simulink model "Lateral"  (R2020a)
settings: Solver=VariableStepAuto  StartTime=0.0  StopTime=5  RelTol=1e-3
settings Model: Creator=hp  LastModifiedBy=hp

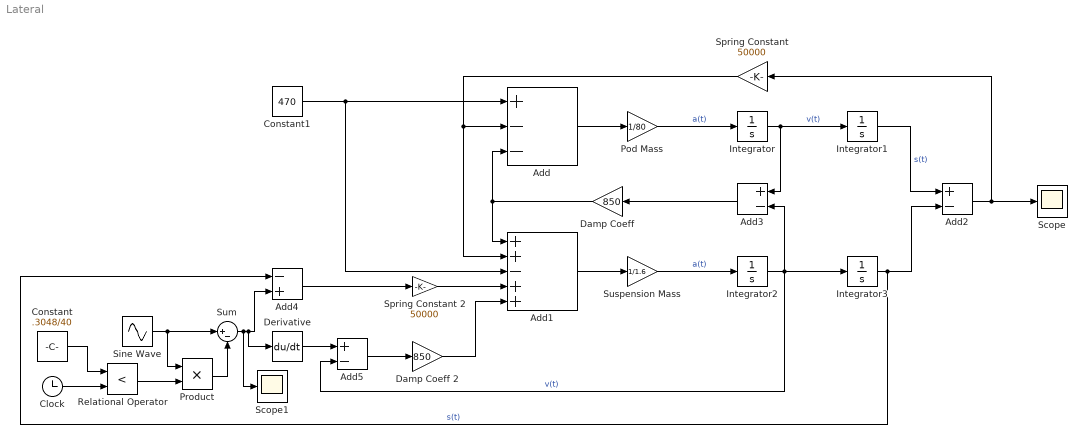
== system Lateral ==
  Add : Sum  Inputs=+--
  Add1 : Sum  Inputs=++-++
  Add2 : Sum  Inputs=+-
  Add3 : Sum  Inputs=+-
  Add4 : Sum  Inputs=-+
  Add5 : Sum  Inputs=+-
  Clock : Clock
  Constant : Constant  Value=.3048/40
  Constant1 : Constant  Value=470
  Damp Coeff : Gain  Gain=850
  Damp Coeff 2 : Gain  Gain=850
  Derivative : Derivative
  Integrator : Integrator  InitialCondition=40
  Integrator1 : Integrator
  Integrator2 : Integrator  InitialCondition=40
  Integrator3 : Integrator
  Pod Mass : Gain  Gain=1/80
  Product : Product
  Relational Operator : RelationalOperator  Operator=<  OutDataTypeStr=boolean  RndMeth=Simplest
  Scope : Scope
  Scope1 : Scope
  Sine Wave : Sin  Amplitude=0.05  Frequency=3.1415926535897/(.3048/40)  SampleTime=0
  Spring Constant : Gain  Gain=50000
  Spring Constant 2 : Gain  Gain=50000
  Sum : Sum  Inputs=|+-
  Suspension Mass : Gain  Gain=1/1.6
  wires:
  Sum/1 -> Scope1/1, Add4/2, Derivative/1
  Add3/1 -> Damp Coeff/1
  Constant/1 -> Relational Operator/1
  Clock/1 -> Relational Operator/2
  Relational Operator/1 -> Product/2
  Add5/1 -> Damp Coeff 2/1
  Integrator/1 -> Add3/1, Integrator1/1  "v(t)"
  Spring Constant/1 -> Add1/2, Add/2
  Add4/1 -> Spring Constant 2/1
  Suspension Mass/1 -> Integrator2/1  "a(t)"
  Spring Constant 2/1 -> Add1/4
  Product/1 -> Sum/2
  Damp Coeff 2/1 -> Add1/5
  Integrator3/1 -> Add2/2, Add4/1  "s(t)"
  Add1/1 -> Suspension Mass/1
  Derivative/1 -> Add5/1
  Damp Coeff/1 -> Add1/1, Add/3
  Sine Wave/1 -> Product/1, Sum/1
  Add2/1 -> Scope/1, Spring Constant/1
  Add/1 -> Pod Mass/1
  Integrator1/1 -> Add2/1  "s(t)"
  Integrator2/1 -> Add5/2, Add3/2, Integrator3/1  "v(t)"
  Constant1/1 -> Add1/3, Add/1
  Pod Mass/1 -> Integrator/1  "a(t)"
